simulink model "cir1_pz1"  (R2024a)
settings: Solver=FixedStepAuto  StartTime=0.0  StopTime=100.0  FixedStep=0.05  RelTol=1e-3
settings Model: Creator=Max  LastModifiedBy=Max

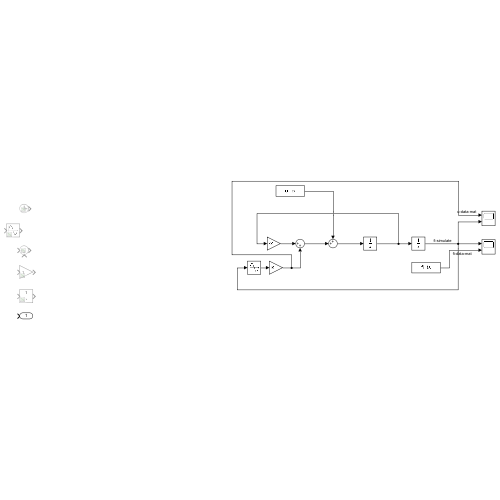
[thumbnail: Simulink's stored preview of the top-level diagram]
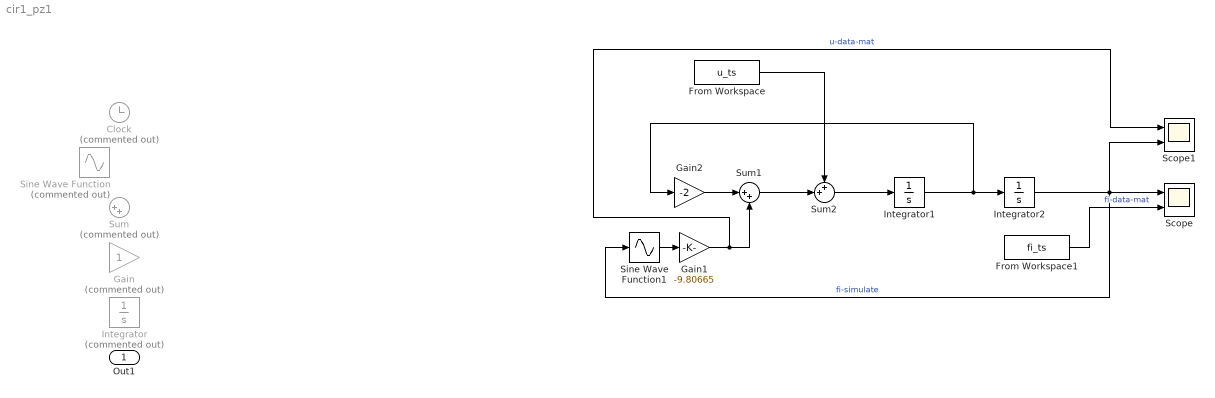
== system cir1_pz1 ==
  Clock : Clock  Commented=on
  From Workspace : FromWorkspace  VariableName=u_ts  SampleTime=0.05
  From Workspace1 : FromWorkspace  VariableName=fi_ts  SampleTime=0.05
  Gain : Gain  Commented=on
  Gain1 : Gain  Gain=-9.80665
  Gain2 : Gain  Gain=-2
  Integrator : Integrator  Commented=on
  Integrator1 : Integrator
  Integrator2 : Integrator
  Scope : Scope  NumInputPorts=2
  Scope1 : Scope  NumInputPorts=2
  Sine Wave Function : Sin  Commented=on  TimeSource=Use external signal  SampleTime=0
  Sine Wave Function1 : Sin  TimeSource=Use external signal  SampleTime=0
  Sum : Sum  Commented=on  Inputs=|++
  Sum1 : Sum  Inputs=|++
  Sum2 : Sum  Inputs=++|
  Out1 : Outport
  wires:
  Integrator1/1 -> Gain2/1, Integrator2/1
  Integrator2/1 -> Scope1/2, Scope/1, Sine Wave Function1/1  "fi-simulate"
  Sine Wave Function1/1 -> Gain1/1
  Gain1/1 -> Scope1/1, Sum1/2  "u-data-mat"
  Gain2/1 -> Sum1/1
  Sum2/1 -> Integrator1/1
  Sum1/1 -> Sum2/2
  From Workspace/1 -> Sum2/1
  From Workspace1/1 -> Scope/2  "fi-data-mat"
